simulink model "SIMULACION"  (R2019b)
settings: Solver=VariableStepAuto  StartTime=0.0  StopTime=200  RelTol=1e-3
undefined symbols (not defined in the file or in its folder): denIN, numIN
libraries: simulink x1
settings Model: Creator=HP  LastModifiedBy=HP

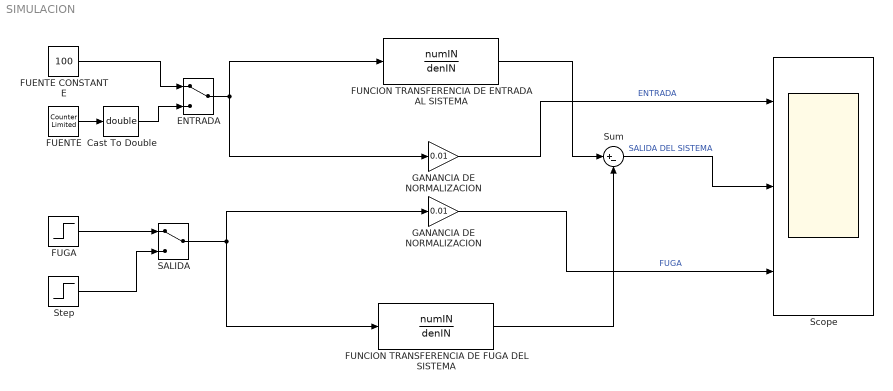
== system SIMULACION ==
  Cast To Double : DataTypeConversion  OutDataTypeStr=double
  ENTRADA : ManualSwitch
  "FUENTE " : simulink/Sources/Counter Limited  uplimit=50  tsamp=2
  FUENTE CONSTANTE : Constant  Value=100
  FUGA : Step  Time=30  After=10  SampleTime=1
  FUNCION TRANSFERENCIA DE ENTRADA AL SISTEMA : TransferFcn  Numerator=numIN  Denominator=denIN
  FUNCION TRANSFERENCIA DE FUGA DEL SISTEMA : TransferFcn  Numerator=numIN  Denominator=denIN
  GANANCIA DE NORMALIZACION : Gain  Gain=0.01
  "GANANCIA DE NORMALIZACION " : Gain  Gain=0.01
  SALIDA : ManualSwitch
  Scope : Scope  NumInputPorts=3
  Step : Step  Time=50  After=15  SampleTime=2
  Sum : Sum  Inputs=|+-
  wires:
  FUNCION TRANSFERENCIA DE ENTRADA AL SISTEMA/1 -> Sum/1
  FUNCION TRANSFERENCIA DE FUGA DEL SISTEMA/1 -> Sum/2
  SALIDA/1 -> "GANANCIA DE NORMALIZACION "/1, FUNCION TRANSFERENCIA DE FUGA DEL SISTEMA/1
  Step/1 -> SALIDA/2
  ENTRADA/1 -> FUNCION TRANSFERENCIA DE ENTRADA AL SISTEMA/1, GANANCIA DE NORMALIZACION/1
  "FUENTE "/1 -> Cast To Double/1
  FUENTE CONSTANTE/1 -> ENTRADA/1
  FUGA/1 -> SALIDA/1
  Cast To Double/1 -> ENTRADA/2
  Sum/1 -> Scope/2  "SALIDA DEL SISTEMA"
  GANANCIA DE NORMALIZACION/1 -> Scope/1  "ENTRADA"
  "GANANCIA DE NORMALIZACION "/1 -> Scope/3  "FUGA"
